simulink model "test_VCT"  (R2014a)
settings: Solver=ode45  StartTime=0.0  StopTime=24*3600  RelTol=1e-3
libraries: refrigeration x1
settings Model: Creator=avenger  LastModifiedBy=avenger
settings OptimizationCC: SimCompilerOptimization=off
settings DebuggingCC: MergeDetectMultiDrivingBlocksExec=error  FrameProcessingCompatibilityMsg=error
settings RTWCC: RTWCompilerOptimization=off

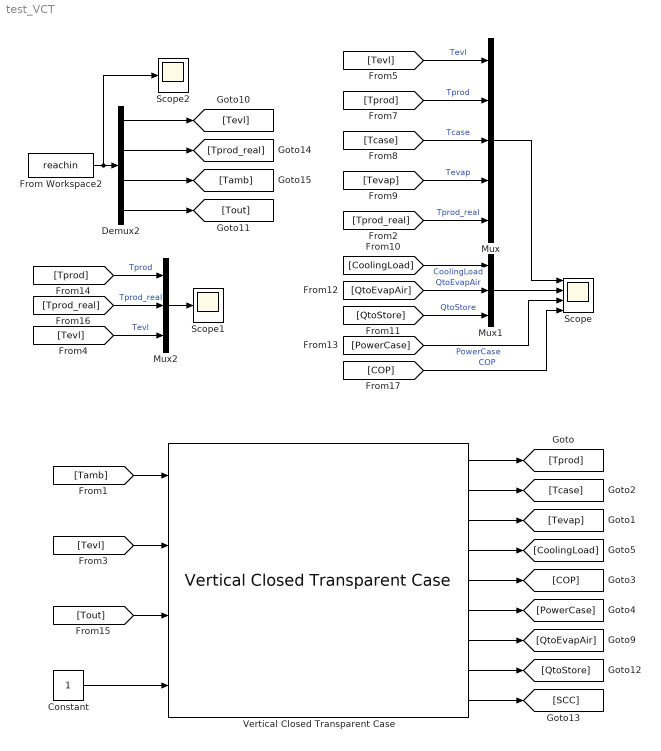
== system test_VCT ==
  Constant : Constant
  Demux2 : Demux
  From Workspace2 : FromWorkspace  VariableName=reachin  SampleTime=0
  Mux : Mux  Inputs=5
  Mux1 : Mux  Inputs=3
  Mux2 : Mux  Inputs=3
  Scope : Scope  NumInputPorts=4
      settings: ShowLegends=on  TimeRange=700000  YMin=-30~-10000~0~-5  YMax=40~10000~60~5
  Scope1 : Scope
      settings: ShowLegends=on  TimeRange=700000  YMin=-25
  Scope2 : Scope
      settings: ShowLegends=on  TimeRange=700000  YMin=-25  SaveName=ScopeData2
  Vertical Closed Transparent Case : refrigeration/Refrigeration/Vertical Closed Transparent Case  Tcase_0=0  Tprod_0=0  Tevap_0=0  Cprod=9.6310e4  Rcase=7.7559e-2  Ccase=9.4247e5  Beta=1.0376e-2  Alpha=3.8101e-2  Gamma=1.2792e-2  RatedLoad=4255  Qinternal=1484  LHR=0.1011  Cevap=150000  p_value=500
  wires:
  Mux/1 -> Scope/1
  [Tevl] -> Mux/1  "Tevl"
  [Tcase] -> Mux/3  "Tcase"
  [Tevap] -> Mux/4  "Tevap"
  [Tprod] -> Mux/2  "Tprod"
  Mux1/1 -> Scope/2
  [QtoEvapAir] -> Mux1/2  "QtoEvapAir"
  [CoolingLoad] -> Mux1/1  "CoolingLoad"
  [PowerCase] -> Scope/3  "PowerCase"
  [QtoStore] -> Mux1/3  "QtoStore"
  Vertical Closed Transparent Case/1 -> [Tprod]
  Vertical Closed Transparent Case/2 -> [Tcase]
  Vertical Closed Transparent Case/3 -> [Tevap]
  Vertical Closed Transparent Case/4 -> [CoolingLoad]
  [Tevl] -> Vertical Closed Transparent Case/2
  [Tout] -> Vertical Closed Transparent Case/3
  [Tamb] -> Vertical Closed Transparent Case/1
  Constant/1 -> Vertical Closed Transparent Case/4
  Vertical Closed Transparent Case/5 -> [COP]
  Vertical Closed Transparent Case/6 -> [PowerCase]
  Vertical Closed Transparent Case/7 -> [QtoEvapAir]
  Vertical Closed Transparent Case/8 -> [QtoStore]
  From Workspace2/1 -> Scope2/1, Demux2/1
  Demux2/1 -> [Tevl]
  Demux2/2 -> [Tprod_real]
  Demux2/3 -> [Tamb]
  Demux2/4 -> [Tout]
  [Tprod_real] -> Mux/5  "Tprod_real"
  [Tprod_real] -> Mux2/2  "Tprod_real"
  [Tprod] -> Mux2/1  "Tprod"
  Mux2/1 -> Scope1/1
  Vertical Closed Transparent Case/9 -> [SCC]
  [COP] -> Scope/4  "COP"
  [Tevl] -> Mux2/3  "Tevl"
